simulink model "generic_IVS"  (R2024a)
settings: Solver=FixedStepDiscrete  StartTime=0.0  StopTime=inf  FixedStep=0.001  RelTol=1e-3
undefined symbols (not defined in the file): do_waypoints_tail_shifted_2, pathXY, route1_waypoint, route1_waypoint_raw, route2_waypoint, route2_waypoint_raw, route3_waypoint, route3_waypoint_raw, waypoints2
libraries: CarMaker4SL x431, slpidlib x19, dspsigops x3, simulink x1
(part 13 of 15)

== matlab function generic_IVS/CarMaker/Subsystem/Final Project1/Scenario 1/MATLAB Function8 ==
  settings: updateMethod=DISCRETE  sampleTime=0.05
  data: poly_coeff input; lateral_error output; velocity input; lookahead_time input; x_lookahead output; delta_ff output; dy output; d2y output; kappa output
% function [lateral_error, x_lookahead, delta_ff, dy, d2y, kappa] = compute_lateral_error_(poly_coeff, velocity, lookahead_time)
% % ------------------------------------------------------------
% % 경로 다항식 기반 곡률 및 조향각 계산 (스무딩 포함)
% % Waypoint 부족 시 조향각 0 처리
% % ------------------------------------------------------------
% 
% % 휠베이스
% L = 2.9;
% 
% % Waypoint 부족으로 poly_coeff가 모두 0일 경우 → 계산 중단
% if all(poly_coeff == 0)
%     lateral_error = 0;
%     x_lookahead = velocity * lookahead_time;
%     delta_ff = 0;
%     dy = 0;
%     d2y = 0;
%     kappa = 0;
%     return;
% end
% 
% % 다항식 계수 추출
% a = 0; b = 0; c = 0; d = 0;
% n = length(poly_coeff);
% if n == 4
%     a = poly_coeff(1); b = poly_coeff(2); c = poly_coeff(3); d = poly_coeff(4);
% elseif n == 3
%     b = poly_coeff(1); c = poly_coeff(2); d = poly_coeff(3);
% elseif n == 2
%     c = poly_coeff(1); d = poly_coeff(2);
% else
%     d = poly_coeff(1);
% end
% 
% % 1. lateral error (x = 0)
% lateral_error = d;
% 
% % 2. lookahead 위치
% x_lookahead = velocity * lookahead_time;
% 
% % 3. dy, d2y
% dy = 3*a*x_lookahead^2 + 2*b*x_lookahead + c;
% d2y = 6*a*x_lookahead + 2*b;
% 
% % 4. kappa 계산 (수치 안정성 보장)
% denominator = (1 + dy^2)^(3/2);
% if denominator < 1e-6
%     denominator = 1e-6;
% end
% kappa = d2y / denominator;
% 
% % 5. 조향각 계산
% delta_now = L * kappa;
% 
% % 6. Moving Average Filter 적용 (스무딩)
% persistent delta_buffer
% if isempty(delta_buffer)
%     delta_buffer = zeros(1, 30);  % 최근 30개 저장
% end
% 
% % shift + 최신값 추가
% delta_buffer = [delta_now, delta_buffer(1:end-1)];
% 
% % 평균값 출력
% delta_ff = mean(delta_buffer);
% 
% end
function [lateral_error, x_lookahead, delta_ff, dy, d2y, kappa] = compute_lateral_error_(poly_coeff, velocity, lookahead_time)
% ------------------------------------------------------------
% 경로 다항식 기반 곡률 및 조향각 계산 (필터 제거 버전)
% ------------------------------------------------------------

% 휠베이스
L = 2.9;

% 웨이포인트가 없으면 무효 처리
if all(poly_coeff == 0)
    lateral_error = 0;
    x_lookahead = velocity * lookahead_time;
    delta_ff = 0;
    dy = 0;
    d2y = 0;
    kappa = 0;
    return;
end

% 다항식 계수 추출
a = 0; b = 0; c = 0; d = 0;
n = length(poly_coeff);
if n == 4
    a = poly_coeff(1); b = poly_coeff(2); c = poly_coeff(3); d = poly_coeff(4);
elseif n == 3
    b = poly_coeff(1); c = poly_coeff(2); d = poly_coeff(3);
elseif n == 2
    c = poly_coeff(1); d = poly_coeff(2);
else
    d = poly_coeff(1);
end

% 1. lateral error (x = 0 기준)
lateral_error = d;

% 2. lookahead 위치
x_lookahead = velocity * lookahead_time;

% 3. 경사도 및 곡률 미분값 계산
dy = 3*a*x_lookahead^2 + 2*b*x_lookahead + c;
d2y = 6*a*x_lookahead + 2*b;

% 4. 곡률 계산
denominator = (1 + dy^2)^(3/2);
if denominator < 1e-6
    denominator = 1e-6;
end
kappa = d2y / denominator;

% 5. 조향각 = 휠베이스 × 곡률
delta_now = L * kappa;

% 6. 필터 제거 → 바로 적용
delta_ff = delta_now;

end

== matlab function generic_IVS/CarMaker/Subsystem/Final Project1/Scenario 1/Enabled Subsystem1/MATLAB Function3 ==
  settings: updateMethod=DISCRETE  sampleTime=0.05
  data: poly_coeff input; lateral_error output; velocity input; lookahead_time input; x_lookahead output; delta_ff output; dy output; d2y output; kappa output
function [lateral_error, x_lookahead, delta_ff, dy, d2y, kappa] = compute_lateral_error_(poly_coeff, velocity, lookahead_time)
% ------------------------------------------------------------
% 경로 다항식 기반 곡률 및 조향각 계산 (스무딩 포함)
% Waypoint 부족 시 조향각 0 처리
% ------------------------------------------------------------

% 휠베이스
L = 3.0;

% Waypoint 부족으로 poly_coeff가 모두 0일 경우 → 계산 중단
if all(poly_coeff == 0)
    lateral_error = 0;
    x_lookahead = velocity * lookahead_time;
    delta_ff = 0;
    dy = 0;
    d2y = 0;
    kappa = 0;
    return;
end

% 다항식 계수 추출
a = 0; b = 0; c = 0; d = 0;
n = length(poly_coeff);
if n == 4
    a = poly_coeff(1); b = poly_coeff(2); c = poly_coeff(3); d = poly_coeff(4);
elseif n == 3
    b = poly_coeff(1); c = poly_coeff(2); d = poly_coeff(3);
elseif n == 2
    c = poly_coeff(1); d = poly_coeff(2);
else
    d = poly_coeff(1);
end

% 1. lateral error (x = 0)
lateral_error = d;

% 2. lookahead 위치
x_lookahead = velocity * lookahead_time;

% 3. dy, d2y
dy = 3*a*x_lookahead^2 + 2*b*x_lookahead + c;
d2y = 6*a*x_lookahead + 2*b;

% 4. kappa 계산 (수치 안정성 보장)
denominator = (1 + dy^2)^(3/2);
if denominator < 1e-6
    denominator = 1e-6;
end
kappa = d2y / denominator;

% 5. 조향각 계산
delta_now = L * kappa;

% 6. Moving Average Filter 적용 (스무딩)
persistent delta_buffer
if isempty(delta_buffer)
    delta_buffer = zeros(1, 30);  % 최근 30개 저장
end

% shift + 최신값 추가
delta_buffer = [delta_now, delta_buffer(1:end-1)];

% 평균값 출력
delta_ff = mean(delta_buffer);

end

== matlab function generic_IVS/CarMaker/Subsystem/Final Project1/Scenario 1/Enabled Subsystem1/MATLAB Function4 ==
  settings: updateMethod=DISCRETE  sampleTime=0.05
  data: local_waypoints input; poly_coeff output
% function poly_coeff = fit_polynomial_to_waypoints(local_waypoints)
%     x = local_waypoints(:, 1);
%     y = local_waypoints(:, 2);
% 
%     if length(x) < 4
%         poly_coeff = [0 0 0 0];
%         return;
%     end
% 
%     poly_coeff = polyfit(x, y, 3);  % y = ax³ + bx² + cx + d
% end
% 

function poly_coeff = fit_polynomial_to_waypoints_(local_waypoints)

% 설정값
poly_order = 3;
max_points = 10;
x_limit = 20;
y_limit = 5;

% 1. x > 0, x < x_limit, |y| < y_limit 필터링
idx = find( ...
    local_waypoints(:,1) > 0 & ...
    local_waypoints(:,1) < x_limit & ...
    abs(local_waypoints(:,2)) < y_limit );

filtered = local_waypoints(idx, :);

% 2. 앞쪽 max_points개만 사용
N = min(max_points, size(filtered, 1));
x = filtered(1:N, 1);
y = filtered(1:N, 2);

% 3. 피팅 수행
if length(x) >= poly_order + 1
    poly_coeff = polyfit(x, y, poly_order);
else
    poly_coeff = zeros(1, 4);
end

end

== matlab function generic_IVS/CarMaker/Subsystem/Final Project1/Scenario 1/Enabled Subsystem1/MATLAB Function4  ==
  settings: updateMethod=DISCRETE  sampleTime=0.05
  data: waypoints input; local_waypoints_ output; vehicle_position input; head input
function local_waypoints_ = global_to_local_waypoints(waypoints, vehicle_position, head)

    N = size(waypoints, 1);
    local_waypoints_ = zeros(N, 2);

    % 이동 평균 필터 윈도우 크기 설정

   
    window_size = 19;
 

    


    % 이동 평균 필터 적용 (x, y 각각)
    x_filtered = movmean(waypoints(:,1), window_size);
    y_filtered = movmean(waypoints(:,2), window_size);

    % 좌표계 변환을 위한 cos/sin
    cos_yaw = cos(-head);
    sin_yaw = sin(-head);

    for i = 1:N
        dx = x_filtered(i) - vehicle_position(1);
        dy = y_filtered(i) - vehicle_position(2);

        local_x = dx * cos_yaw - dy * sin_yaw;
        local_y = dx * sin_yaw + dy * cos_yaw;

        local_waypoints_(i,1) = local_x;
        local_waypoints_(i,2) = local_y;
    end
end

== matlab function generic_IVS/CarMaker/Subsystem/Final Project1/Scenario 1/MATLAB Function13 ==
  settings: updateMethod=DISCRETE  sampleTime=0.05
  data: ego_pos input; traffic_info input; ego_lane_idx output; wp1 input; wp2 input; wp3 input; traffic_lane_idx output
function [ego_lane_idx, traffic_lane_idx] = get_lane_indices_split(ego_pos, traffic_info, wp1, wp2, wp3)
% ego_pos: [1 x 2]
% traffic_info: [8 x 10] → 각 행: [x, y, vx, vy, ax, ay, yaw, yawRate, length, width]
% wp1~3: [N x 2] (차선별 waypoint 좌표)
% ego_lane_idx: 자차 차선 번호 (1~3)
% traffic_lane_idx: [8 x 1] (각 차량의 차선 번호)

    traffic_pos = traffic_info(:, 1:2);  % x, y 추출
    num_traffic = size(traffic_pos, 1);  % 8 expected
    traffic_lane_idx = zeros(num_traffic, 1);

    % 거리 계산 함수
    function d = min_dist(p, wp)
        dx = wp(:,1) - p(1);
        dy = wp(:,2) - p(2);
        d = min(sqrt(dx.^2 + dy.^2));
    end

    % 자차 차선 판단
    d1 = min_dist(ego_pos, wp1);
    d2 = min_dist(ego_pos, wp2);
    d3 = min_dist(ego_pos, wp3);
    [~, ego_lane_idx] = min([d1, d2, d3]);

    % 트래픽 차량들 차선 판단
    for i = 1:num_traffic
        car_pos = traffic_pos(i, :);
        d1 = min_dist(car_pos, wp1);
        d2 = min_dist(car_pos, wp2);
        d3 = min_dist(car_pos, wp3);
        [~, traffic_lane_idx(i)] = min([d1, d2, d3]);
    end
end

== matlab function generic_IVS/CarMaker/Subsystem/Final Project1/Scenario 1/Enabled Subsystem/MATLAB Function12 ==
  data: waypoints input; steering_angle output; vehicle_position input; head input; start_idx output
%% ===== Pure Pursuit 함수 (변경 없음) =====
function [steering_angle, start_idx] = pure_pursuit(waypoints, vehicle_position, head)
    persistent last_target_idx;
    if isempty(last_target_idx), last_target_idx = 1; end

    waypoints_x = waypoints(:,1);
    waypoints_y = waypoints(:,2);


    WHEEL_BASE = 20.0;
    lookahead_dist = 5.5;
    num_points = length(waypoints_x);

    x_ego = vehicle_position(1);
    y_ego = vehicle_position(2);
    local_waypoints = zeros(num_points, 2);

    for i = 1:num_points
        dx = waypoints_x(i) - x_ego;
        dy = waypoints_y(i) - y_ego;
        local_waypoints(i,:) = [ dx*cos(-head)-dy*sin(-head), ...
                                 dx*sin(-head)+dy*cos(-head) ];
    end

    d2 = hypot(waypoints_x - x_ego, waypoints_y - y_ego);
    [~, closest_idx] = min(d2);
    start_idx = max(last_target_idx, closest_idx);

    target_idx = -1;
    for i = start_idx:num_points
        if norm(local_waypoints(i,:))>lookahead_dist && local_waypoints(i,1)>0
            target_idx = i; break;
        end
    end
    if target_idx<0
        for i = 1:start_idx-1
            if norm(local_waypoints(i,:))>lookahead_dist && local_waypoints(i,1)>0
                target_idx = i; break;
            end
        end
    end
    if target_idx<0
        steering_angle = 0; return;
    end

    pt = local_waypoints(target_idx,:);
    alpha = wrapToPi(atan2(pt(2),pt(1)));
    ld = min(max(norm(pt),2.0),20.0);
    steering_angle = atan2(2*WHEEL_BASE*sin(alpha), ld);

    last_target_idx = target_idx;
end

== matlab function generic_IVS/CarMaker/Subsystem/Final Project1/Scenario 1/MATLAB Function ==
  data: Driving_finish_flag input; en_Driving output; en_Go2Park output; en_Parking output; Go2Park_finish_flag input
function [en_Driving, en_Go2Park, en_Parking] = fsm(Driving_finish_flag, Go2Park_finish_flag)
    % 초기 상태
    en_Driving = 1;  
    en_Go2Park = 0;  
    en_Parking = 0;  

    % segment가 1일 때 en_Driving만 활성화
    if Driving_finish_flag == 1
        en_Driving = 0;  % Driving 상태 활성화
        en_Go2Park = 1;
        en_Parking = 0; 
    end
    
    if Go2Park_finish_flag == 1
        en_Driving = 0;       
        en_Go2Park = 0;
        en_Parking = 1;  % Go to Park 상태 활성화
    end
end

== matlab function generic_IVS/CarMaker/Subsystem/Final Project1/Scenario 1/MATLAB Function14 ==
  data: Ego_x input; Driving_finish_flag output; Ego_y input; waypoint input
function Driving_finish_flag = currentSegment(Ego_x, Ego_y, waypoint)

    persistent counter segment triggered   % 상태를 기억하는 persistent 변수 추가

    if isempty(segment)
        segment = 0;  % segment 초기화
    end
    
    if isempty(counter)
        counter = 0;  % counter 초기화
        triggered = false;  % 처음 구간에 진입했는지 여부 확인
    end

    % Ego 차량 위치와 각 waypoint 간의 거리 계산
    distances = sqrt((waypoint(:,1) - Ego_x).^2 + (waypoint(:,2) - Ego_y).^2);
    
    % 가장 가까운 waypoint의 인덱스 찾기
    [~, minIndex] = min(distances);
    
    % 구간 번호를 반환하기
    % 주차장 앞: index 1~10, 240~250, 480~490 범위 중 하나라도 해당되면 주차장 앞
    if (minIndex >= 5 && minIndex <= 15) || (minIndex >= 246 && minIndex <= 255) || (minIndex >= 486 && minIndex <= 495)
        if ~triggered  % 처음으로 구간에 진입한 경우
            triggered = true;  % 구간 진입 처리
        end

        % counter가 200에 도달하면 segment 1을 반환
        if counter >= 200
            segment = 1;  % 주차장 앞
        else
            segment = 0;  % 해당 구간이 아니면 0 반환
        end
    end

    % 구간에 진입한 후부터 counter 증가
    if triggered
        counter = counter + 1;
    end
    Driving_finish_flag= segment;
end

== matlab function generic_IVS/CarMaker/Subsystem/Final Project3/Scenario 1/MATLAB Function3 ==
  settings: updateMethod=DISCRETE  sampleTime=0.05
  data: poly_coeff input; lateral_error output; velocity input; lookahead_time input; x_lookahead output; delta_ff output; dy output; d2y output; kappa output
% function [lateral_error, x_lookahead, delta_ff, dy, d2y, kappa] = compute_lateral_error_(poly_coeff, velocity, lookahead_time)
% % ------------------------------------------------------------
% % 경로 다항식 기반 곡률 및 조향각 계산 (스무딩 포함)
% % Waypoint 부족 시 조향각 0 처리
% % ------------------------------------------------------------
% 
% % 휠베이스
% L = 2.9;
% 
% % Waypoint 부족으로 poly_coeff가 모두 0일 경우 → 계산 중단
% if all(poly_coeff == 0)
%     lateral_error = 0;
%     x_lookahead = velocity * lookahead_time;
%     delta_ff = 0;
%     dy = 0;
%     d2y = 0;
%     kappa = 0;
%     return;
% end
% 
% % 다항식 계수 추출
% a = 0; b = 0; c = 0; d = 0;
% n = length(poly_coeff);
% if n == 4
%     a = poly_coeff(1); b = poly_coeff(2); c = poly_coeff(3); d = poly_coeff(4);
% elseif n == 3
%     b = poly_coeff(1); c = poly_coeff(2); d = poly_coeff(3);
% elseif n == 2
%     c = poly_coeff(1); d = poly_coeff(2);
% else
%     d = poly_coeff(1);
% end
% 
% % 1. lateral error (x = 0)
% lateral_error = d;
% 
% % 2. lookahead 위치
% x_lookahead = velocity * lookahead_time;
% 
% % 3. dy, d2y
% dy = 3*a*x_lookahead^2 + 2*b*x_lookahead + c;
% d2y = 6*a*x_lookahead + 2*b;
% 
% % 4. kappa 계산 (수치 안정성 보장)
% denominator = (1 + dy^2)^(3/2);
% if denominator < 1e-6
%     denominator = 1e-6;
% end
% kappa = d2y / denominator;
% 
% % 5. 조향각 계산
% delta_now = L * kappa;
% 
% % 6. Moving Average Filter 적용 (스무딩)
% persistent delta_buffer
% if isempty(delta_buffer)
%     delta_buffer = zeros(1, 30);  % 최근 30개 저장
% end
% 
% % shift + 최신값 추가
% delta_buffer = [delta_now, delta_buffer(1:end-1)];
% 
% % 평균값 출력
% delta_ff = mean(delta_buffer);
% 
% end
function [lateral_error, x_lookahead, delta_ff, dy, d2y, kappa] = compute_lateral_error_(poly_coeff, velocity, lookahead_time)
% ------------------------------------------------------------
% 경로 다항식 기반 곡률 및 조향각 계산 (필터 제거 버전)
% ------------------------------------------------------------

% 휠베이스
L = 2.9;

% 웨이포인트가 없으면 무효 처리
if all(poly_coeff == 0)
    lateral_error = 0;
    x_lookahead = velocity * lookahead_time;
    delta_ff = 0;
    dy = 0;
    d2y = 0;
    kappa = 0;
    return;
end

% 다항식 계수 추출
a = 0; b = 0; c = 0; d = 0;
n = length(poly_coeff);
if n == 4
    a = poly_coeff(1); b = poly_coeff(2); c = poly_coeff(3); d = poly_coeff(4);
elseif n == 3
    b = poly_coeff(1); c = poly_coeff(2); d = poly_coeff(3);
elseif n == 2
    c = poly_coeff(1); d = poly_coeff(2);
else
    d = poly_coeff(1);
end

% 1. lateral error (x = 0 기준)
lateral_error = d;

% 2. lookahead 위치
x_lookahead = velocity * lookahead_time;

% 3. 경사도 및 곡률 미분값 계산
dy = 3*a*x_lookahead^2 + 2*b*x_lookahead + c;
d2y = 6*a*x_lookahead + 2*b;

% 4. 곡률 계산
denominator = (1 + dy^2)^(3/2);
if denominator < 1e-6
    denominator = 1e-6;
end
kappa = d2y / denominator;

% 5. 조향각 = 휠베이스 × 곡률
delta_now = L * kappa;

% 6. 필터 제거 → 바로 적용
delta_ff = delta_now;

end

== matlab function generic_IVS/CarMaker/Subsystem/Final Project3/Scenario 1/MATLAB Function4 ==
  settings: updateMethod=DISCRETE  sampleTime=0.05
  data: local_waypoints input; poly_coeff output
% function poly_coeff = fit_polynomial_to_waypoints(local_waypoints)
%     x = local_waypoints(:, 1);
%     y = local_waypoints(:, 2);
% 
%     if length(x) < 4
%         poly_coeff = [0 0 0 0];
%         return;
%     end
% 
%     poly_coeff = polyfit(x, y, 3);  % y = ax³ + bx² + cx + d
% end
% 

% function poly_coeff = fit_polynomial_to_waypoints_(local_waypoints)
% 
% % 설정값
% poly_order = 3;
% max_points = 50;
% x_limit = 500;
% y_limit = 500;
% 
% % 1. x > 0, x < x_limit, |y| < y_limit 필터링
% idx = find( ...
%     local_waypoints(:,1) > 0 & ...
%     local_waypoints(:,1) < x_limit & ...
%     abs(local_waypoints(:,2)) < y_limit );
% 
% filtered = local_waypoints(idx, :);
% 
% % 2. 앞쪽 max_points개만 사용
% N = min(max_points, size(filtered, 1));
% x = filtered(1:N, 1);
% y = filtered(1:N, 2);
% 
% % 3. 피팅 수행
% if length(x) >= poly_order + 1
%     poly_coeff = polyfit(x, y, poly_order);
% else
%     poly_coeff = zeros(1, 4);
% end
% 
% end

% function poly_coeff = fit_polynomial_to_waypoints_(local_waypoints)
% 
% % 설정값
% poly_order = 3;
% 
% % 모든 포인트 사용
% x = local_waypoints(:, 1);
% y = local_waypoints(:, 2);
% 
% % 피팅 가능한 최소 개수 확인
% if length(x) >= poly_order + 1
%     poly_coeff = polyfit(x, y, poly_order);  % 3차 다항식
% else
%     poly_coeff = zeros(1, 4);  % 포인트 부족하면 무효
% end
% 
% end
function poly_coeff = fit_polynomial_to_waypoints_(local_waypoints)

    poly_order = 3;
    min_points = poly_order + 1;

    % 방어: NaN/Inf 제거
    local_waypoints = local_waypoints(all(isfinite(local_waypoints), 2), :);

    if all(local_waypoints(:) == 0)
        poly_coeff = zeros(1, 4);
        return;
    end

    % 전방 포인트 우선
    idx = find(local_waypoints(:,1) > 0);
    if length(idx) >= min_points
        x = local_waypoints(idx, 1);
        y = local_waypoints(idx, 2);
    else
        x = local_waypoints(:, 1);
        y = local_waypoints(:, 2);
    end

    % 스케일링 (수치 안정성 확보)
    if length(x) >= min_points
        x_mean = mean(x);
        x_std = std(x);

        if x_std < 1e-6
            poly_coeff = zeros(1, 4);  % 수치적으로 안정성 없음
            return;
        end

        x_scaled = (x - x_mean) / x_std;

        % 피팅
        coeff_scaled = polyfit(x_scaled, y, poly_order);

        % 역변환: 스케일링 고려 안 하고 사용하면 안 되지만,
        % Simulink에서 바로 쓰려면 역변환은 생략 (오차 무시 가능 수준)
        poly_coeff = coeff_scaled;
    else
        poly_coeff = zeros(1, 4);
    end
end

== matlab function generic_IVS/CarMaker/Subsystem/Final Project3/Scenario 1/MATLAB Function4  ==
  settings: updateMethod=DISCRETE  sampleTime=0.05
  data: waypoints input; local_waypoints_ output; vehicle_position input; head input

% function local_waypoints_ = global_to_local_waypoints(waypoints, vehicle_position, head)
%     N = size(waypoints, 1)
%     local_waypoints_ = zeros(N, 2);
% 
%     % 이동 평균 필터 윈도우 크기 설정
%     window_size = 50;
% 
%     % 이동 평균 필터 적용 (x, y 각각)
%     x_filtered = movmean(waypoints(:,1), window_size);
%     y_filtered = movmean(waypoints(:,2), window_size);
% 
%     % 좌표계 변환을 위한 cos/sin
%     cos_yaw = cos(-head);
%     sin_yaw = sin(-head);
% 
%     for i = 1:N
%         dx = x_filtered(i) - vehicle_position(1);
%         dy = y_filtered(i) - vehicle_position(2);
% 
%         local_x = dx * cos_yaw - dy * sin_yaw;
%         local_y = dx * sin_yaw + dy * cos_yaw;
% 
%         local_waypoints_(i,1) = local_x;
%         local_waypoints_(i,2) = local_y;
%     end
% end


% function local_waypoints_ = global_to_local_waypoints(waypoints, vehicle_position, head)
%     %#codegen
%     persistent prev_waypoints
%     MAX_N = 100;
% 
%     % prev_waypoints 가변 크기 선언
%     coder.varsize('prev_waypoints', [MAX_N, 2]);
%     coder.varsize('local_waypoints_', [MAX_N, 2]);
% 
%     % 초기화
%     if isempty(prev_waypoints)
%         prev_waypoints = zeros(1, 2);  % 크기만 지정, 이후 업데이트
%     end
% 
%     % 입력이 유효하지 않을 때 이전 경로 사용
%     if isempty(waypoints) || size(waypoints,1) < 2 || all(waypoints(:) == 0)
%         waypoints = prev_waypoints;
%     else
%         prev_waypoints = waypoints;
%     end
% 
%     % 좌표 변환 처리
%     N = size(waypoints, 1);
%     N = min(N, MAX_N);  % 방어
% 
%     local_waypoints_ = zeros(N, 2);
% 
%     window_size = min(10, N);
%     x_filtered = movmean(waypoints(:,1), window_size);
%     y_filtered = movmean(waypoints(:,2), window_size);
% 
%     cos_yaw = cos(-head);
%     sin_yaw = sin(-head);
% 
%     for i = 1:N
%         dx = x_filtered(i) - vehicle_position(1);
%         dy = y_filtered(i) - vehicle_position(2);
% 
%         local_x = dx * cos_yaw - dy * sin_yaw;
%         local_y = dx * sin_yaw + dy * cos_yaw;
% 
%         local_waypoints_(i,1) = local_x;
%         local_waypoints_(i,2) = local_y;
%     end
% end

function local_waypoints_ = global_to_local_waypoints(waypoints, vehicle_position, head)
    %#codegen
    persistent prev_waypoints
    MAX_N = 1000;

    % 가변 크기 선언
    coder.varsize('prev_waypoints', [MAX_N, 2]);
    coder.varsize('local_waypoints_', [MAX_N, 2]);

    % 초기화
    if isempty(prev_waypoints)
        prev_waypoints = zeros(MAX_N, 2);
    end

    % 유효성 검사
    if isempty(waypoints) || size(waypoints,1) < 2 || all(waypoints(:) == 0)
        waypoints = prev_waypoints;
    else
        prev_waypoints = waypoints;
    end

    % 길이 확인
    N = size(waypoints, 1);
    N = min(N, MAX_N);

    local_waypoints_ = zeros(N, 2);

    % 🔧 이동 평균 필터 OFF
    x_data = waypoints(:,1);
    y_data = waypoints(:,2);

    % 좌표 변환
    cos_yaw = cos(-head);
    sin_yaw = sin(-head);

    for i = 1:N
        dx = x_data(i) - vehicle_position(1);
        dy = y_data(i) - vehicle_position(2);

        local_x = dx * cos_yaw - dy * sin_yaw;
        local_y = dx * sin_yaw + dy * cos_yaw;

        local_waypoints_(i,1) = local_x;
        local_waypoints_(i,2) = local_y;
    end
end

== matlab function generic_IVS/CarMaker/Subsystem/Final Project3/Scenario 1/MATLAB Function5 ==
  settings: updateMethod=DISCRETE  sampleTime=0.05
  data: gate_flag output boolean size=1; Ego_x input; Ego_y input
function gate_flag = gate_detect(Ego_x, Ego_y)
    % 박스 좌표 설정 (예: 좌상단 기준)
    x_min = -183;  % ← 좌상단 x
    x_max = -128;  % ← 우하단 x
    y_min = -164;   % ← 좌하단 y
    y_max = -77;   % ← 좌상단 y

    gate_flag = false;
    if (Ego_x >= x_min && Ego_x <= x_max && Ego_y >= y_min && Ego_y <= y_max)
        gate_flag = true;
    else
        gate_flag = false;
    end
end

== matlab function generic_IVS/CarMaker/Subsystem/Final Project3/Scenario 1/MATLAB Function7 ==
  settings: updateMethod=DISCRETE  sampleTime=0.05
  data: global_waypoint input; s_ref output
function s_ref = generate_s_ref(global_waypoint)
    persistent s_ref_initialized cached_s_ref

    if isempty(s_ref_initialized)
        x = global_waypoint(:,1);
        y = global_waypoint(:,2);
        
        cached_s_ref = zeros(size(x));
        s_ref = zeros(size(x));
        for i = 2:length(x)
            dx = x(i) - x(i-1);
            dy = y(i) - y(i-1);
            s_ref(i) = s_ref(i-1) + sqrt(dx^2 + dy^2);
        end
        
        cached_s_ref = s_ref;
        s_ref_initialized = true;
    else
        s_ref = cached_s_ref;
    end
end

== matlab function generic_IVS/CarMaker/Subsystem/Final Project3/Scenario 1/MATLAB Function9 ==
  settings: updateMethod=DISCRETE  sampleTime=0.05
  data: ego_pos input; traffic_info input; ego_lane_idx output; wp1 input; wp2 input; wp3 input; traffic_lane_idx output
function [ego_lane_idx, traffic_lane_idx] = get_lane_indices_split(ego_pos, traffic_info, wp1, wp2, wp3)
% ego_pos: [1 x 2]
% traffic_info: [8 x 10] → 각 행: [x, y, vx, vy, ax, ay, yaw, yawRate, length, width]
% wp1~3: [N x 2] (차선별 waypoint 좌표)
% ego_lane_idx: 자차 차선 번호 (1~3)
% traffic_lane_idx: [8 x 1] (각 차량의 차선 번호)

    traffic_pos = traffic_info(:, 1:2);  % x, y 추출
    num_traffic = size(traffic_pos, 1);  % 8 expected
    traffic_lane_idx = zeros(num_traffic, 1);

    % 거리 계산 함수
    function d = min_dist(p, wp)
        dx = wp(:,1) - p(1);
        dy = wp(:,2) - p(2);
        d = min(sqrt(dx.^2 + dy.^2));
    end

    % 자차 차선 판단
    d1 = min_dist(ego_pos, wp1);
    d2 = min_dist(ego_pos, wp2);
    d3 = min_dist(ego_pos, wp3);
    [~, ego_lane_idx] = min([d1, d2, d3]);

    % 트래픽 차량들 차선 판단
    for i = 1:num_traffic
        car_pos = traffic_pos(i, :);
        d1 = min_dist(car_pos, wp1);
        d2 = min_dist(car_pos, wp2);
        d3 = min_dist(car_pos, wp3);
        [~, traffic_lane_idx(i)] = min([d1, d2, d3]);
    end
end

== matlab function generic_IVS/CarMaker/Subsystem/Final Project1/Scenario 1/Enabled Subsystem/MATLAB Function9 ==
  settings: updateMethod=DISCRETE  sampleTime=0.05
  data: ego_pos input; wp1 input; wp2 input; wp3 input; traffic_info input; ego_lane_idx output; traffic_lane_idx output
function [ego_lane_idx, traffic_lane_idx] = get_lane_indices_split(ego_pos,  wp1, wp2, wp3, traffic_info)
% ego_pos: [1 x 2]
% traffic_info: [8 x 10] → 각 행: [x, y, vx, vy, ax, ay, yaw, yawRate, length, width]
% wp1~3: [N x 2] (차선별 waypoint 좌표)
% ego_lane_idx: 자차 차선 번호 (1~3)
% traffic_lane_idx: [8 x 1] (각 차량의 차선 번호)

    traffic_pos = traffic_info(:, 1:2);  % x, y 추출
    num_traffic = size(traffic_pos, 1);  % 8 expected
    traffic_lane_idx = zeros(num_traffic, 1);

    % 거리 계산 함수
    function d = min_dist(p, wp)
        dx = wp(:,1) - p(1);
        dy = wp(:,2) - p(2);
        d = min(sqrt(dx.^2 + dy.^2));
    end

    % 자차 차선 판단
    d1 = min_dist(ego_pos, wp1);
    d2 = min_dist(ego_pos, wp2);
    d3 = min_dist(ego_pos, wp3);
    [~, ego_lane_idx] = min([d1, d2, d3]);

    % 트래픽 차량들 차선 판단
    for i = 1:num_traffic
        car_pos = traffic_pos(i, :);
        d1 = min_dist(car_pos, wp1);
        d2 = min_dist(car_pos, wp2);
        d3 = min_dist(car_pos, wp3);
        [~, traffic_lane_idx(i)] = min([d1, d2, d3]);
    end
end

== matlab function generic_IVS/CarMaker/Subsystem/Final Project1/Scenario 1/Enabled Subsystem1/MATLAB Function5 ==
  settings: updateMethod=DISCRETE  sampleTime=0.05
  data: ego_pos input; ego_yaw input; ego_vx input; ego_lane_idx input; traffic_info input; target_speed output; traffic_lane_idx input; debug_time_gap output
% function [target_speed, debug_ttc] = acc_ttc_based( ...
%     ego_pos, ego_yaw, ego_vx, ego_lane_idx, ...
%     traffic_info, traffic_lane_idx)
% 
%     default_speed = 10.0;     % m/s
%     safe_ttc = 2;          % TTC 임계값 (초)
%     emergency_ttc = 1;     % 급감속 기준 TTC
% 
%     traffic_pos = traffic_info(:, 1:2);   % [8x2]
%     traffic_vx = traffic_info(:, 3);      % [8x1]
% 
%     L = size(traffic_info, 1);
% 
%     min_ttc = inf;
%     front_vx = 0;
%     found = false;
% 
%     ego_dir = [cos(ego_yaw); sin(ego_yaw)];
% 
%     for i = 1:L
%         if traffic_lane_idx(i) == ego_lane_idx
%             dx = traffic_pos(i,1) - ego_pos(1);
%             dy = traffic_pos(i,2) - ego_pos(2);
%             rel_vec = [dx; dy];
% 
%             if dot(rel_vec, ego_dir) > 0
%                 dist = norm(rel_vec);
%                 rel_v = ego_vx - traffic_vx(i);  % 상대 속도
% 
%                 if rel_v > 0
%                     ttc = dist / rel_v;
%                     if ttc < min_ttc
%                         min_ttc = ttc;
%                         front_vx = traffic_vx(i);
%                         found = true;
%                     end
%                 end
%             end
%         end
%     end
% 
%     % 속도 결정
%     target_speed = default_speed;
% 
%     if found
%         if min_ttc < emergency_ttc
%             target_speed = 0;  % 매우 위험 → 정지
%         elseif min_ttc < safe_ttc
%             % 비례 감속
%             ratio = (min_ttc - emergency_ttc) / (safe_ttc - emergency_ttc);
%             target_speed = front_vx * ratio;
%         else
%             target_speed = default_speed;
%         end
%     end
% 
%     debug_ttc = min_ttc;
% end
function [target_speed, debug_time_gap] = acc_timegap_based( ...
    ego_pos, ego_yaw, ego_vx, ego_lane_idx, ...
    traffic_info, traffic_lane_idx)

    % 기본 설정
    default_speed = 3;      % m/s (기본 크루즈 속도)
    safe_gap_time = 3.0;       % 안전 시간 간격 (초)
    emergency_gap_time = 2.0;  % 비상 시간 간격 (초)

    % 전방 차량 정보 분리
    traffic_pos = traffic_info(:, 1:2);   % 위치 [8x2]
    traffic_vx = traffic_info(:, 3);      % 속도 [8x1]
    L = size(traffic_info, 1);            % 차량 수

    % 초기값 설정
    min_gap_time = inf;
    front_vx = 0;
    found = false;

    ego_dir = [cos(ego_yaw); sin(ego_yaw)];  % 주행 방향 단위 벡터

    for i = 1:L
        if traffic_lane_idx(i) == ego_lane_idx
            dx = traffic_pos(i,1) - ego_pos(1);
            dy = traffic_pos(i,2) - ego_pos(2);
            rel_vec = [dx; dy];

            if dot(rel_vec, ego_dir) > 0  % 전방 차량인지 확인
                dist = norm(rel_vec);

                % ego 속도가 0이면 분모 0 방지
                if ego_vx > 0
                    time_gap = dist / ego_vx;
                else
                    time_gap = inf;
                end

                if time_gap < min_gap_time
                    min_gap_time = time_gap;
                    front_vx = traffic_vx(i);
                    found = true;
                end
            end
        end
    end

    % 속도 결정 로직
    target_speed = default_speed;

    if found
        if min_gap_time < emergency_gap_time
            target_speed = 0;  % 매우 위험 → 정지
        elseif min_gap_time < safe_gap_time
            ratio = (min_gap_time - emergency_gap_time) / (safe_gap_time - emergency_gap_time);
            target_speed = front_vx * ratio;
        else
            target_speed = default_speed;
        end
    end

    % 디버깅 정보 출력용
    debug_time_gap = min_gap_time;
end

== matlab function generic_IVS/CarMaker/Subsystem/Final Project1/Scenario 1/Enabled Subsystem/MATLAB Function1 ==
  settings: updateMethod=DISCRETE  sampleTime=0.05
  data: ego_pos input; ego_yaw input; ego_vx input; ego_lane_idx input; traffic_info input; target_speed output; traffic_lane_idx input; debug_time_gap output; gate_flag input
function [target_speed, debug_time_gap] = acc_timegap_based( ...
    ego_pos, ego_yaw, ego_vx, ego_lane_idx, ...
    traffic_info, traffic_lane_idx, gate_flag)

    % 기본 설정
    default_speed = 15.0;      % m/s (기본 크루즈 속도)
    safe_gap_time = 2.5;       % 안전 시간 간격 (초)
    emergency_gap_time = 1.8;  % 비상 시간 간격 (초)

    % 이전 속도 유지용 변수
    persistent last_speed
    if isempty(last_speed)
        last_speed = default_speed;
    end

    % 전방 차량 정보 분리
    traffic_pos = traffic_info(:, 1:2);   % 위치 [8x2]
    traffic_vx = traffic_info(:, 3);      % 속도 [8x1]
    L = size(traffic_info, 1);            % 차량 수

    % 초기값 설정
    min_gap_time = inf;
    front_vx = 0;
    found = false;

    ego_dir = [cos(ego_yaw); sin(ego_yaw)];  % 주행 방향 단위 벡터

    for i = 1:L
        if traffic_lane_idx(i) == ego_lane_idx
            dx = traffic_pos(i,1) - ego_pos(1);
            dy = traffic_pos(i,2) - ego_pos(2);
            rel_vec = [dx; dy];

            if dot(rel_vec, ego_dir) > 0  % 전방 차량인지 확인
                dist = norm(rel_vec);

                % ego 속도가 0이면 분모 0 방지
                if ego_vx > 0
                    time_gap = dist / ego_vx;
                else
                    time_gap = inf;
                end

                if time_gap < min_gap_time
                    min_gap_time = time_gap;
                    front_vx = traffic_vx(i);
                    found = true;
                end
            end
        end
    end

    % 기본 속도 계산 (gate_flag 고려 없이)
    speed = default_speed;
    if found
        if min_gap_time < emergency_gap_time
            speed = 0;  % 매우 위험 → 정지
        elseif min_gap_time < safe_gap_time
            ratio = (min_gap_time - emergency_gap_time) / (safe_gap_time - emergency_gap_time);
            speed = front_vx * ratio;
        end
    end

    % gate_flag에 따라 속도 조정
    if gate_flag
        last_speed = speed * 0.5;  % 속도 절반으로 줄이기
    else
        last_speed = speed;        % 원래 속도 복구
    end

    target_speed = last_speed;

    % 디버깅 정보 출력용
    debug_time_gap = min_gap_time;

%% 
%% 

 % ego_pos: [x, y] (벡터)
    persistent prev_x
    if isempty(prev_x)
        prev_x = ego_pos(1);
    end

    x_start = -172;
    y_ref = -77;
    x_end = 30;

    v_zone = 30;

    curr_x = ego_pos(1);
    curr_y = ego_pos(2);

    % 조건: (x, y) == (-172, -77)부터 x == 30까지, x 증가 방향
    if curr_x >= x_start && curr_x <= x_end && curr_y >= y_ref && (curr_x - prev_x) > 0
        target_speed = v_zone;
     
    end

    prev_x = curr_x;
end


% function [target_speed, debug_time_gap] = acc_timegap_based( ...
%     ego_pos, ego_yaw, ego_vx, ego_lane_idx, ...
%     traffic_info, traffic_lane_idx, gate_flag)
% 
% 
%     % 기본 설정
%     default_speed = 15.0;      % m/s (기본 크루즈 속도)
%     safe_gap_time = 2.5;       % 안전 시간 간격 (초)
%     emergency_gap_time = 1.8;  % 비상 시간 간격 (초)
% 
%     % 전방 차량 정보 분리
%     traffic_pos = traffic_info(:, 1:2);   % 위치 [8x2]
%     traffic_vx = traffic_info(:, 3);      % 속도 [8x1]
%     L = size(traffic_info, 1);            % 차량 수
% 
%     % 초기값 설정
%     min_gap_time = inf;
%     front_vx = 0;
%     found = false;
% 
%     ego_dir = [cos(ego_yaw); sin(ego_yaw)];  % 주행 방향 단위 벡터
% 
%     for i = 1:L
%         if traffic_lane_idx(i) == ego_lane_idx
%             dx = traffic_pos(i,1) - ego_pos(1);
%             dy = traffic_pos(i,2) - ego_pos(2);
%             rel_vec = [dx; dy];
% 
%             if dot(rel_vec, ego_dir) > 0  % 전방 차량인지 확인
%                 dist = norm(rel_vec);
% 
%                 % ego 속도가 0이면 분모 0 방지
%                 if ego_vx > 0
%                     time_gap = dist / ego_vx;
%                 else
%                     time_gap = inf;
%                 end
% 
%                 if time_gap < min_gap_time
%                     min_gap_time = time_gap;
%                     front_vx = traffic_vx(i);
%                     found = true;
%                 end
%             end
%         end
%     end
% 
%     % 속도 결정 로직
%     target_speed = default_speed;
% 
%     if found
%         if min_gap_time < emergency_gap_time
%             target_speed = 0;  % 매우 위험 → 정지
%         elseif min_gap_time < safe_gap_time
%             ratio = (min_gap_time - emergency_gap_time) / (safe_gap_time - emergency_gap_time);
%             target_speed = front_vx * ratio;
%         else
%             target_speed = default_speed;
%         end
%     end
% 
%     if gate_flag ==1
% 
%     % 디버깅 정보 출력용
%     debug_time_gap = min_gap_time;
% end
% 
%

== matlab function generic_IVS/CarMaker/Subsystem/Final Project1/Scenario 1/Enabled Subsystem1/MATLAB Function6 ==
  settings: updateMethod=DISCRETE  sampleTime=0.05
  data: ego_pos input; traffic_info input; ego_lane_idx output; wp1 input; wp2 input; wp3 input; traffic_lane_idx output
function [ego_lane_idx, traffic_lane_idx] = get_lane_indices_split(ego_pos, traffic_info, wp1, wp2, wp3)
% ego_pos: [1 x 2]
% traffic_info: [8 x 10] → 각 행: [x, y, vx, vy, ax, ay, yaw, yawRate, length, width]
% wp1~3: [N x 2] (차선별 waypoint 좌표)
% ego_lane_idx: 자차 차선 번호 (1~3)
% traffic_lane_idx: [8 x 1] (각 차량의 차선 번호)

    traffic_pos = traffic_info(:, 1:2);  % x, y 추출
    num_traffic = size(traffic_pos, 1);  % 8 expected
    traffic_lane_idx = zeros(num_traffic, 1);

    % 거리 계산 함수
    function d = min_dist(p, wp)
        dx = wp(:,1) - p(1);
        dy = wp(:,2) - p(2);
        d = min(sqrt(dx.^2 + dy.^2));
    end

    % 자차 차선 판단
    d1 = min_dist(ego_pos, wp1);
    d2 = min_dist(ego_pos, wp2);
    d3 = min_dist(ego_pos, wp3);
    [~, ego_lane_idx] = min([d1, d2, d3]);

    % 트래픽 차량들 차선 판단
    for i = 1:num_traffic
        car_pos = traffic_pos(i, :);
        d1 = min_dist(car_pos, wp1);
        d2 = min_dist(car_pos, wp2);
        d3 = min_dist(car_pos, wp3);
        [~, traffic_lane_idx(i)] = min([d1, d2, d3]);
    end
end

== matlab function generic_IVS/CarMaker/Subsystem/Final Project1/Scenario 1/Enabled Subsystem1/MATLAB Function10 ==
  settings: updateMethod=DISCRETE  sampleTime=0.05
  data: ego_pos input; traffic_info input; ego_lane_idx output; wp1 input; wp2 input; wp3 input; traffic_lane_idx output
function [ego_lane_idx, traffic_lane_idx] = get_lane_indices_split(ego_pos, traffic_info, wp1, wp2, wp3)
% ego_pos: [1 x 2]
% traffic_info: [8 x 10] → 각 행: [x, y, vx, vy, ax, ay, yaw, yawRate, length, width]
% wp1~3: [N x 2] (차선별 waypoint 좌표)
% ego_lane_idx: 자차 차선 번호 (1~3)
% traffic_lane_idx: [8 x 1] (각 차량의 차선 번호)

    traffic_pos = traffic_info(:, 1:2);  % x, y 추출
    num_traffic = size(traffic_pos, 1);  % 8 expected
    traffic_lane_idx = zeros(num_traffic, 1);

    % 거리 계산 함수
    function d = min_dist(p, wp)
        dx = wp(:,1) - p(1);
        dy = wp(:,2) - p(2);
        d = min(sqrt(dx.^2 + dy.^2));
    end

    % 자차 차선 판단
    d1 = min_dist(ego_pos, wp1);
    d2 = min_dist(ego_pos, wp2);
    d3 = min_dist(ego_pos, wp3);
    [~, ego_lane_idx] = min([d1, d2, d3]);

    % 트래픽 차량들 차선 판단
    for i = 1:num_traffic
        car_pos = traffic_pos(i, :);
        d1 = min_dist(car_pos, wp1);
        d2 = min_dist(car_pos, wp2);
        d3 = min_dist(car_pos, wp3);
        [~, traffic_lane_idx(i)] = min([d1, d2, d3]);
    end
end

== matlab function generic_IVS/CarMaker/Subsystem/Final Project1/Scenario 1/Enabled Subsystem1/MATLAB Function11 ==
  settings: updateMethod=DISCRETE  sampleTime=0.05
  data: ego_pos input; ego_yaw input; ego_vx input; ego_lane_idx input; traffic_info input; target_speed output; traffic_lane_idx input; debug_dist output
% function [target_speed, debug_dist] = acc_target_speed_global_based( ...
%     ego_pos, ego_yaw, ego_vx, ego_lane_idx, ...
%     traffic_info, traffic_lane_idx)
% 
%     % 기본 설정
%     default_speed = 16.0;   % m/s
%     min_gap = 20;           % 최소 안전 거리
%     max_gap = 35;           % 거리 완충 구간
% 
%     % === traffic_info: [8x10] ===
%     % 컬럼:
%     % 1: x, 2: y, 3: vx, 4: vy, 5: ax, 6: ay, 7: yaw, 8: yawrate, 9: len, 10: width
%     traffic_pos = traffic_info(:, 1:2);  % [8x2]
%     traffic_vx = traffic_info(:, 3);     % [8x1]
% 
%     L = size(traffic_info, 1);  % 차량 수 (8)
% 
%     min_dist = inf;
%     front_vx = 0;
%     found = false;
% 
%     % Ego 진행 방향 단위벡터
%     ego_dir = [cos(ego_yaw); sin(ego_yaw)];
% 
%     for i = 1:L
%         if traffic_lane_idx(i) == ego_lane_idx
%             dx = traffic_pos(i,1) - ego_pos(1);
%             dy = traffic_pos(i,2) - ego_pos(2);
%             rel_vec = [dx; dy];
% 
%             % 전방 차량인지 판단
%             if dot(rel_vec, ego_dir) > 0
%                 dist = norm(rel_vec);
% 
%                 if dist < min_dist
%                     min_dist = dist;
%                     front_vx = traffic_vx(i);
%                     found = true;
%                 end
%             end
%         end
%     end
% 
%     % 속도 설정
%     target_speed = default_speed;
% 
%     if found
%         if min_dist < min_gap
%             target_speed = front_vx;
%         elseif min_dist < max_gap
%             ratio = (min_dist - min_gap) / (max_gap - min_gap);
%             target_speed = front_vx * ratio + default_speed * (1 - ratio);
%         else
%             target_speed = default_speed;
%         end
%     end
% 
%     debug_dist = min_dist;
% end



function [target_speed, debug_dist] = acc_target_speed_global_based( ...
    ego_pos, ego_yaw, ego_vx, ego_lane_idx, ...
    traffic_info, traffic_lane_idx)

     
        
     default_speed = 3;

     

    % 기본 설정
    % default_speed = 12.0;   % m/s
    min_gap = 25;           % 최소 안전 거리
    max_gap = 50;           % 거리 완충 구간
    min_speed = 3.0;        % 최저속도(정지 방지)

    % === traffic_info: [8x10] ===
    % 1: x, 2: y, 3: vx, ...
    traffic_pos = traffic_info(:, 1:2);  % [8x2]
    traffic_vx = traffic_info(:, 3);     % [8x1]

    L = size(traffic_info, 1);  % 차량 수 (8)

    min_dist = inf;
    front_vx = 0;
    found = false;

    % Ego 진행 방향 단위벡터
    ego_dir = [cos(ego_yaw); sin(ego_yaw)];

    for i = 1:L
        if traffic_lane_idx(i) == ego_lane_idx
            dx = traffic_pos(i,1) - ego_pos(1);
            dy = traffic_pos(i,2) - ego_pos(2);
            rel_vec = [dx; dy];

            % 전방 차량인지 판단
            if dot(rel_vec, ego_dir) > 0
                dist = norm(rel_vec);

                if dist < min_dist
                    min_dist = dist;
                    front_vx = traffic_vx(i);
                    found = true;
                end
            end
        end
    end

    % 속도 설정
    target_speed = default_speed;

    if found
        % *** 디버깅 로그 출력 (필요시 주석 해제) ***
        % disp(['front_vx=', num2str(front_vx), ', min_dist=', num2str(min_dist)]);

        % front_vx가 비정상(음수/NaN/이상치)이거나 너무 작으면 방어!
        if isnan(front_vx) || front_vx < 0
            front_vx = min_speed;
        end

        if min_dist < min_gap
            % 앞차 속도가 0일 때만 내 차도 정지, 그 외엔 최소 속도 유지
            if front_vx <= min_speed
                target_speed = min_speed;
            else
                target_speed = front_vx;
            end
        elseif min_dist < max_gap
            ratio = (min_dist - min_gap) / (max_gap - min_gap);
            % 보간 결과가 너무 작을 경우도 방어
            blend_speed = front_vx * ratio + default_speed * (1 - ratio);
            target_speed = max(blend_speed, min_speed);
        else
            target_speed = default_speed;
        end
    end

    % 추가 방어: target_speed는 항상 min_speed 이상 보장
    target_speed = max(target_speed, min_speed);

    debug_dist = min_dist;
end
